simulink model "model"  (R2019a)
settings: Solver=ode4  StartTime=0.0  StopTime=0.1  FixedStep=0.0001  RelTol=1e-5
values from neighbouring files (symbols this model uses):
  a11 = -(i_n*(r_v+r_j))/(N*P_n)    (= -36.6666666667)    [lab3.m]
  a12 = -c_e*w_n/N    (= -483.333333333)    [lab3.m]
  a13 = U_sn/(N*P_n)    (= 366.666666667)    [lab3.m]
  a21 = a11    (= -36.6666666667)    [lab3.m]
  a22 = a12    (= -483.333333333)    [lab3.m]
  a23 = a13    (= 366.666666667)    [lab3.m]
  a31 = c_m*P_n*i_n/(J*w_n)    (= 11.5)    [lab3.m]
  a32 = -M_sn/(J*w_n)    (= -47)    [lab3.m]
  Q2 = [-0.381 0 2.292 0 0.3415]    [lab3.m]
undefined symbols (not defined in the file or in its folder): Mc, Uc, X, x0
settings Model: Creator=khanh  LastModifiedBy=ogure
settings DataIOCC: ReturnWorkspaceOutputs=off
settings DebuggingCC: ArithmeticOperatorsInVariantConditions=warning
settings SFSimCC: SimUseLocalCustomCode=off
settings RTWCC: RTWUseLocalCustomCode=off
settings CodeAppCC: StateflowObjectComments=on

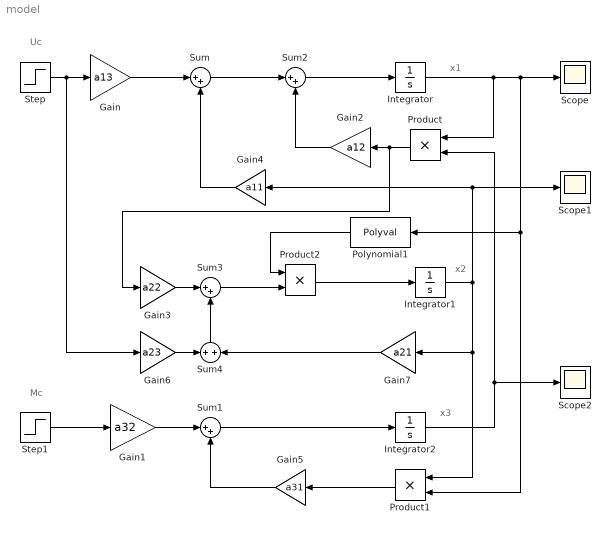
== system model ==
  note: Mc
  note: Uc
  note: x3
  note: x2
  note: x1
  Gain : Gain  Gain=a13
  Gain1 : Gain  Gain=a32
  Gain2 : Gain  Gain=a12
  Gain3 : Gain  Gain=a22
  Gain4 : Gain  Gain=a11
  Gain5 : Gain  Gain=a31
  Gain6 : Gain  Gain=a23
  Gain7 : Gain  Gain=a21
  Integrator : Integrator  InitialCondition=x0(1)+X(1)
  Integrator1 : Integrator  InitialCondition=x0(2)+X(2)
  Integrator2 : Integrator  InitialCondition=x0(3)+X(3)
  Polynomial1 : Polyval  Coefs=[ Q2(1),Q2(2),Q2(3), Q2(4), Q2(5) ]
  Product : Product
  Product1 : Product
  Product2 : Product
  Scope : Scope
  Scope1 : Scope
  Scope2 : Scope
  Step : Step  Time=0  Before=1  After=Uc+1  SampleTime=0
  Step1 : Step  Time=0  Before=1  After=Mc+1  SampleTime=0
  Sum{,1..3} (4 alike) : Sum  Inputs=|++
  Sum4 : Sum  Inputs=+|+
  wires:
  Step/1 -> Gain6/1, Gain/1
  Step1/1 -> Gain1/1
  Gain/1 -> Sum/1
  Sum/1 -> Sum2/1
  Integrator2/1 -> Scope2/1, Product/2
  Gain2/1 -> Sum2/2
  Gain4/1 -> Sum/2
  Gain1/1 -> Sum1/1
  Product1/1 -> Gain5/1
  Gain5/1 -> Sum1/2
  Sum1/1 -> Integrator2/1
  Integrator1/1 -> Gain7/1, Product1/1, Gain4/1, Scope1/1
  Sum2/1 -> Integrator/1
  Integrator/1 -> Polynomial1/1, Product1/2, Scope/1, Product/1
  Product/1 -> Gain3/1, Gain2/1
  Gain3/1 -> Sum3/1
  Gain7/1 -> Sum4/2
  Gain6/1 -> Sum4/1
  Sum4/1 -> Sum3/2
  Product2/1 -> Integrator1/1
  Polynomial1/1 -> Product2/1
  Sum3/1 -> Product2/2
